simulink model "Task1"  (R2025a)
settings: Solver=VariableStepAuto  StartTime=0.0  StopTime=10.0  RelTol=1e-3
settings Model: Creator=LOQ  LastModifiedBy=LOQ

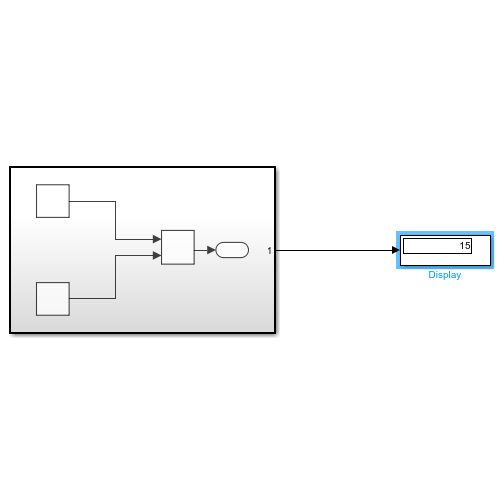
[thumbnail: Simulink's stored preview of the top-level diagram]
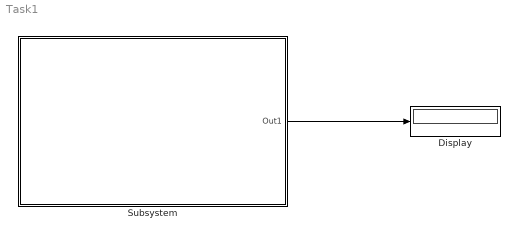
== system Task1 ==
  Display : Display
  Subsystem : Subsystem  TreatAsAtomicUnit=on
  wires:
  Subsystem/1(Out1) -> Display/1

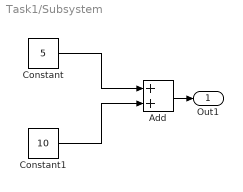
== system Task1/Subsystem ==
  Add : Sum
  Constant : Constant  Value=5
  Constant1 : Constant  Value=10
  Out1 : Outport
  wires:
  Constant/1 -> Add/1
  Constant1/1 -> Add/2
  Add/1 -> Out1/1
